simulink library "CryoDetLibCMB"  (R2016b)
(part 9 of 12)

      settings: infoedit=<html>Valid operands: CONCAT, P, C, PCIN, P>>17, PCIN>>17, CARRYIN, CARRYCASCIN, ACIN, A, BCIN,B<br><br>Valid operators: +, -, *, ()<br><br>Valid functions: RNDSIMPLE, RNDSYM<br><br>Instructions are case insensitive and tolerate spaces.</html>
  Delay{1,3,5,8} (4 alike) : xbsIndex_r4/Delay  rst=off  infoeditControl=Selection of Reset will increase slice count due to use of real FFs and instead of SRLs  en=off  latency=4  reg_retiming=on  dbl_ovrd=off  block_type=delay
  Delay2 : xbsIndex_r4/Delay  rst=off  infoeditControl=Selection of Reset will increase slice count due to use of real FFs and instead of SRLs  en=off  latency=5  reg_retiming=on  dbl_ovrd=off  block_type=delay
  Delay4 : xbsIndex_r4/Delay  rst=off  infoeditControl=Selection of Reset will increase slice count due to use of real FFs and instead of SRLs  en=off  latency=3  reg_retiming=on  dbl_ovrd=off  block_type=delay
  Delay6 : xbsIndex_r4/Delay  rst=off  infoeditControl=Selection of Reset will increase slice count due to use of real FFs and instead of SRLs  en=off  latency=1  reg_retiming=on  dbl_ovrd=off  block_type=delay
  Delay7 : xbsIndex_r4/Delay  rst=off  infoeditControl=Selection of Reset will increase slice count due to use of real FFs and instead of SRLs  en=off  latency=1  reg_retiming=on  dbl_ovrd=off  block_type=delay
  Delay9 : xbsIndex_r4/Delay  rst=off  infoeditControl=Selection of Reset will increase slice count due to use of real FFs and instead of SRLs  en=off  latency=3  reg_retiming=on  dbl_ovrd=off  block_type=delay
  Reinterpret : xbsIndex_r4/Reinterpret  force_arith_type=on  arith_type=Unsigned  force_bin_pt=on  bin_pt=0  block_type=reinterpret
  Reinterpret1 : xbsIndex_r4/Reinterpret  force_arith_type=on  arith_type="Signed  (2's comp)"  force_bin_pt=on  bin_pt=10  block_type=reinterpret
  Subsystem : Subsystem
  Terminator : Terminator
  sign_extend : xbsIndex_r4/Convert  gui_display_data_type=Fixed-point  arith_type="Signed  (2's comp)"  n_bits=18  bin_pt=15  float_type=Single  exp_bits=8  fraction_bits=24  quantization=Truncate  overflow=Wrap  en=off  latency=0  pipeline=off  dbl_ovrd=off  block_type=convert
  sign_extend1 : xbsIndex_r4/Convert  gui_display_data_type=Fixed-point  arith_type="Signed  (2's comp)"  n_bits=24  bin_pt=23  float_type=Single  exp_bits=8  fraction_bits=24  quantization=Truncate  overflow=Saturate  en=off  latency=1  pipeline=off  dbl_ovrd=off  block_type=convert
  valid_o : Outport
  dF_Q : Outport  Port=2
  ch_early_o : Outport  Port=3
  ch_o : Outport  Port=4
  wires:
  Reinterpret1/1 -> "DSP48 Macro 3.0 "/2
  "DSP48 Macro 3.0 "/1 -> sign_extend1/1
  sign_extend1/1 -> dF_Q/1
  sign_extend/1 -> Delay7/1
  AddSub/1 -> sign_extend/1
  Delay7/1 -> "CORDIC 6.0 "/6
  "CORDIC 6.0 "/4 -> Delay6/1  "ch"
  Delay6/1 -> Delay8/1, ch_early_o/1
  Delay5/1 -> "CORDIC 6.0 "/7
  Delay3/1 -> Reinterpret/1
  ref phase/1 -> AddSub/2
  etaPhase/1 -> AddSub/1
  "CORDIC 6.0 "/5 -> Reinterpret1/1  "etaMag"
  Reinterpret/1 -> "CORDIC 6.0 "/4
  Delay2/1 -> valid_o/1
  "CORDIC 6.0 "/1 -> Delay2/1
  Delay1/1 -> "CORDIC 6.0 "/1, "CORDIC 6.0 "/5
  valid/1 -> Delay1/1
  ch/1 -> Delay5/1
  etaMag/1 -> Delay3/1
  "CORDIC 6.0 "/2 -> "DSP48 Macro 3.0 "/1  "Q"
  Q/1 -> Delay4/1
  I/1 -> Delay9/1
  Delay4/1 -> Subsystem/2(Q)
  Delay9/1 -> Subsystem/3(I)
  Subsystem/2(Out2) -> "CORDIC 6.0 "/3
  Subsystem/1(Out1) -> "CORDIC 6.0 "/2
  r_IQ_swap_sel/1 -> Subsystem/1(sel)
  "CORDIC 6.0 "/3 -> Terminator/1  "I"
  Delay8/1 -> ch_o/1
